simulink model "sim3_laboratorium"  (R2023b)
settings: Solver=FixedStepAuto  StartTime=0.0  StopTime=30  FixedStep=0.001  RelTol=1e-3
values from neighbouring files (symbols this model uses):
  deltay = 1    [laboratorium4.m]
  denominator = [ 1, 3, 3, 1 ]    [laboratorium4.m]
  Kr = kp(i)    [laboratorium4.m]
  nominator = ( 1 )    (= 1)    [laboratorium4.m]
  y0 = 0    [laboratorium4.m]
  y_time = 0    [laboratorium4.m]
settings Model: Creator=student  LastModifiedBy=tomasz
settings SolverCC: AlgebraicLoopSolver=TrustRegion
settings DebuggingCC: UnconnectedInputMsg=warning  UnconnectedOutputMsg=warning  UnconnectedLineMsg=warning
settings ModelReferenceCC: EnableRefExpFcnMdlSchedulingChecks=on
settings RTWCC: DLArmComputeVersion=19.05

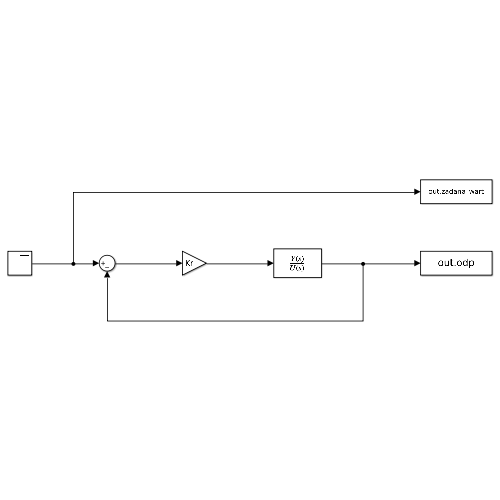
[thumbnail: Simulink's stored preview of the top-level diagram]
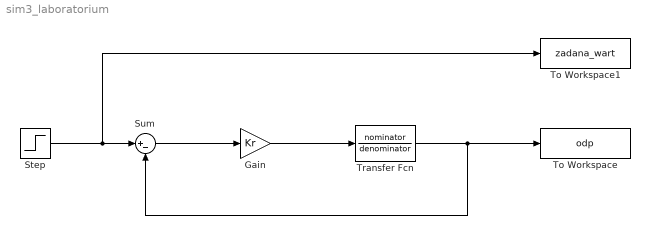
== system sim3_laboratorium ==
  Gain : Gain  Gain=Kr
  Step : Step  Time=y_time  Before=y0  After=y0 + deltay  SampleTime=0
  Sum : Sum  Inputs=|+-
  To Workspace : ToWorkspace  VariableName=odp  SampleTime=-1
      settings: Save2DSignal=2-D array (concatenate along first dimension)
  To Workspace1 : ToWorkspace  VariableName=zadana_wart  SampleTime=-1
      settings: Save2DSignal=2-D array (concatenate along first dimension)
  Transfer Fcn : TransferFcn  Numerator=nominator  Denominator=denominator
  wires:
  Step/1 -> To Workspace1/1, Sum/1
  Gain/1 -> Transfer Fcn/1
  Transfer Fcn/1 -> To Workspace/1, Sum/2
  Sum/1 -> Gain/1
